simulink library "lib_transmission"  (Simulink 4.1.1)
undefined symbols (not defined in the file or in its folder): fc_map_spd, fc_max_trq, fc_spd_scale, fc_trq_scale, fd_inertia, fd_loss, fd_ratio, gb_inertia, gb_loss_const, gb_loss_input_spd_coeff, gb_loss_input_trq_coeff, gb_loss_output_spd_coeff, gb_loss_output_trq_coeff, gb_map_spd_out, gb_map_trq_in, gb_map_trq_out, gb_ratio, gb_spd_scale, gb_trq_scale, htc_inertia, htc_k_adv, htc_k_adv_coast, htc_max_coast_tr, htc_min_coast_tr, htc_sr, htc_sr_coast, htc_tr, htc_tr_coast, mc_map_spd, mc_max_trq, mc_overtrq_factor, mc_spd_scale, mc_trq_scale, tc_loss, tc_mc_to_fc_ratio, tx_eff_map, tx_map_spd, tx_map_trq, tx_pg_r, tx_pg_s, vc_idle_spd, vc_launch_spd
libraries: lib_transmission x2
(part 1 of 3)
settings Model: LastModifiedBy=tmarkel
settings Model: ModifiedComment=|
  | tmarkel -- Fri Sep 20 16:05:52 2002 -- Version 1.102
  | modified Pout/Pin calc block - moved !=0 check to before bombproof block; value after bombproof is never zero
  | 
  | there are still some issues with this calculation to be resolved at a later date
settings Model: ModifiedHistory=|
  | tmarkel -- Fri Sep 20 16:05:52 2002 -- Version 1.102
  | modified Pout/Pin calc block - moved !=0 check to before bombproof block; value after bombproof is never zero
  | 
  | there are still some issues with this calculation to be resolved at a later date
  | 
  | 
  | tmarkel -- Fri Sep 20 14:16:55 2002 -- Version 1.101
  | changed t loss when tx_eff=0 to be the total torque in request
  | 
  | abrooker -- Fri May 24 14:07:33 2002 -- Version 1.100
  | 
  | mokeefe -- Thu Apr 18 08:38:43 2002 -- Version 1.99
  | saving the model:
  | o "without the model browser open"
  | o with only top-level screen visible
  | o with "fit to view" enabled
  | o with "status bar" off and "toolbar" off
  | o with "prompt to update model history with each save" on

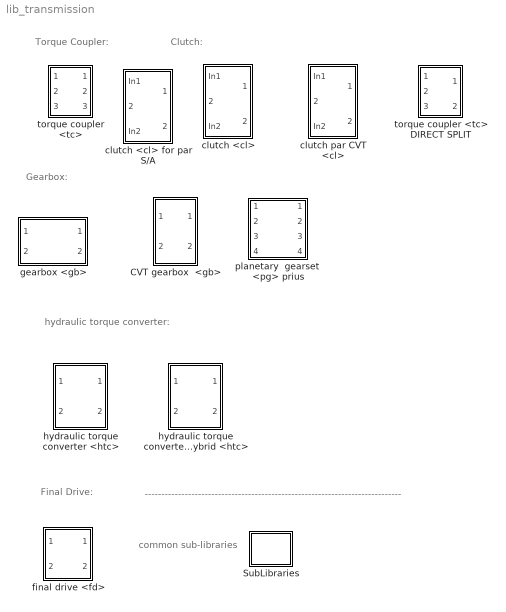
== system lib_transmission ==
  note: Torque Coupler:
  note: Gearbox:
  note: Clutch:
  note: hydraulic torque converter:
  note: Final Drive:
  note: -----------------------------------------------------------------------------
  note: common
      | sub-libraries
  CVT gearbox  <gb> : Subsystem
      settings: RTWFcnNameOpts=Auto  RTWFileNameOpts=Auto
  SubLibraries : Subsystem
      settings: RTWFcnNameOpts=Auto  RTWFileNameOpts=Auto
  clutch <cl> : Subsystem  mask(Clutch){slip_spd=vc_launch_spd, maxtrq=max(fc_max_trq)*fc_trq_scale}
      mask prompts: slip_spd "Input shaft speed when clutch slips (rad/s):"; maxtrq "Maximum torque clutch can transmit:"
      mask help: Clutch for use with ADVISOR 2
      settings: RTWFcnNameOpts=Auto  RTWFileNameOpts=Auto
      mask Help:
      | First input is req'd clutch output torque and speed, muxed together.
      | Second input is clutch state, with 1 => disengaged, 2 => slipping, and 3=> engaged.
      | Third input is available clutch input torque and limited clutch input speed.
      | First output is req'd clutch input torque and speed, muxed together.
      | Second output is available clutch output torque and limited clutch output speed.
      | The logic implemented by this block is as follows:
      |           IF (clutch is disengaged) THEN (req'd input torque=0), (req'd input speed=req'd output speed (the engine control is responsible for computing correct engine spin-down speed)), (avail. output torque=0), (limited output speed=req'd output speed)
      |           IF (clutch is slipping) THEN (req'd input torque=req'd output torque), (req'd input speed=user-defined slip speed), (avail. output torque=avail. input torque), (limited output speed=req'd output speed)
      |           IF (clutch is engaged) THEN (req'd input torque=req'd output torque), (req'd input speed=req'd output speed), (avail. output torque=avail. input torque), (limited output speed=limited input speed)
      | 
      | The clutch will transmit no more than its maximum torque as driving or braking torque.
      mask Display: image(imread('bdi_cl.jpg'))
  clutch <cl> for par S/A : Subsystem  mask(Clutch){slip_spd=vc_launch_spd, maxtrq=max(fc_max_trq)*fc_trq_scale+max(mc_max_trq)*mc_overtrq_factor*mc_trq_scale}
      mask prompts: slip_spd "Input shaft speed when clutch slips (rad/s):"; maxtrq "Maximum torque clutch can transmit:"
      mask help: Clutch for use with ADVISOR 2
      settings: RTWFcnNameOpts=Auto  RTWFileNameOpts=Auto
      mask Help:
      | First input is req'd clutch output torque and speed, muxed together.
      | Second input is clutch state, with 1 => disengaged, 2 => slipping, and 3=> engaged.
      | Third input is available clutch input torque and limited clutch input speed.
      | First output is req'd clutch input torque and speed, muxed together.
      | Second output is available clutch output torque and limited clutch output speed.
      | The logic implemented by this block is as follows:
      |           IF (clutch is disengaged) THEN (req'd input torque=0), (req'd input speed=req'd output speed (the engine control is responsible for computing correct engine spin-down speed)), (avail. output torque=0), (limited output speed=req'd output speed)
      |           IF (clutch is slipping) THEN (req'd input torque=req'd output torque), (req'd input speed=user-defined slip speed), (avail. output torque=avail. input torque), (limited output speed=req'd output speed)
      |           IF (clutch is engaged) THEN (req'd input torque=req'd output torque), (req'd input speed=req'd output speed), (avail. output torque=avail. input torque), (limited output speed=limited input speed)
      | 
      | The clutch will transmit no more than its maximum torque as driving or braking torque.
      mask Display: image(imread('bdi_cl.jpg'))
  clutch par CVT <cl> : Subsystem  mask(Clutch){slip_spd=vc_launch_spd, maxtrq=max(fc_max_trq)*fc_trq_scale+max(mc_max_trq)*mc_trq_scale*mc_overtrq_factor}
      mask prompts: slip_spd "Input shaft speed when clutch slips (rad/s):"; maxtrq "Maximum torque clutch can transmit:"
      mask help: Clutch for use with ADVISOR 2
      settings: RTWFcnNameOpts=Auto  RTWFileNameOpts=Auto
      mask Help:
      | First input is req'd clutch output torque and speed, muxed together.
      | Second input is clutch state, with 1 => disengaged, 2 => slipping, and 3=> engaged.
      | Third input is available clutch input torque and limited clutch input speed.
      | First output is req'd clutch input torque and speed, muxed together.
      | Second output is available clutch output torque and limited clutch output speed.
      | The logic implemented by this block is as follows:
      |           IF (clutch is disengaged) THEN (req'd input torque=0), (req'd input speed=req'd output speed (the engine control is responsible for computing correct engine spin-down speed)), (avail. output torque=0), (limited output speed=req'd output speed)
      |           IF (clutch is slipping) THEN (req'd input torque=req'd output torque), (req'd input speed=user-defined slip speed), (avail. output torque=avail. input torque), (limited output speed=req'd output speed)
      |           IF (clutch is engaged) THEN (req'd input torque=req'd output torque), (req'd input speed=req'd output speed), (avail. output torque=avail. input torque), (limited output speed=limited input speed)
      | 
      | The clutch will transmit no more than its maximum torque as driving or braking torque.
      mask Display: image(imread('bdi_cl.jpg'))
  final drive <fd> : Subsystem
      settings: RTWFcnNameOpts=Auto  RTWFileNameOpts=Auto
      mask Display: image(imread('bdi_fd.jpg'))
  gearbox <gb> : Subsystem
      settings: RTWFcnNameOpts=Auto  RTWFileNameOpts=Auto
      mask Display: image(imread('bdi_gb.jpg'))
  hydraulic torque converter <htc> : Subsystem
      settings: RTWFcnNameOpts=Auto  RTWFileNameOpts=Auto
      mask Display: image(imread('bdi_htc.jpg'))
  hydraulic torque converter for  parallel hybrid <htc> : Subsystem
      settings: RTWFcnNameOpts=Auto  RTWFileNameOpts=Auto
      mask Display: image(imread('bdi_htc.jpg'))
  planetary  gearset  <pg> prius : Subsystem
      settings: RTWFcnNameOpts=Auto  RTWFileNameOpts=Auto
      mask Display: image(imread('bdi_psplit.jpg'))
  torque coupler <tc> : Subsystem
      settings: RTWFcnNameOpts=Auto  RTWFileNameOpts=Auto
      mask Display: image(imread('bdi_tc.jpg'))
  torque coupler <tc> DIRECT SPLIT : Subsystem
      settings: RTWFcnNameOpts=Auto  RTWFileNameOpts=Auto
      mask Display: image(imread('bdi_tc.jpg'))

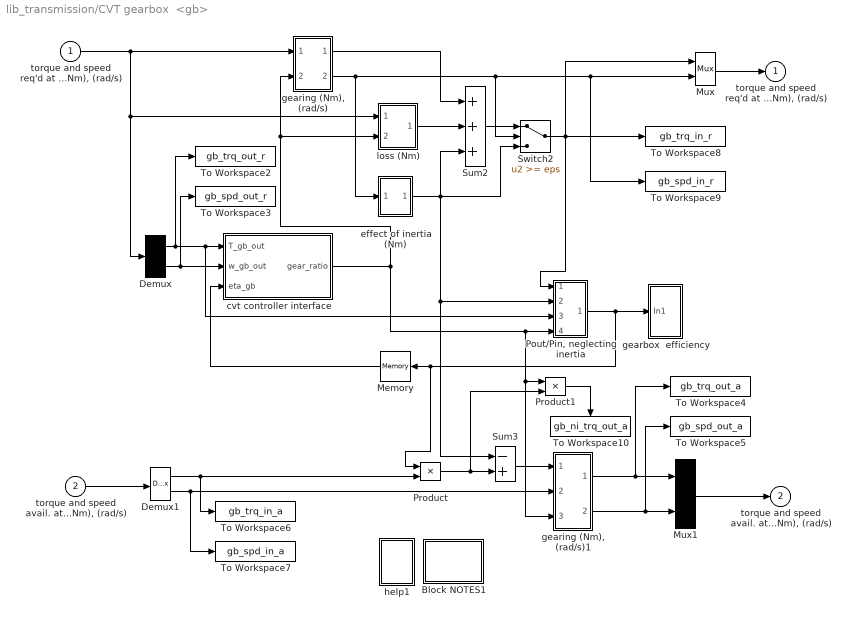
== system lib_transmission/CVT gearbox  <gb> ==
  "torque and speed req'd at output side of cvt (Nm), (rad/s)" : Inport  Port=1  LatchInput=off
  "torque and speed avail. at input side of cvt (Nm), (rad/s)" : Inport  Port=2  LatchInput=off
  Block NOTES1 : Subsystem
      settings: RTWFcnNameOpts=Auto  RTWFileNameOpts=Auto
      mask Display: disp('Block\nNOTES')
  Demux : Demux  Outputs=2  BusSelectionMode=off
  Demux1 : Demux  Outputs=2  BusSelectionMode=off
  Memory : Memory  Orientation=left  X0=0.9  InheritSampleTime=off
      settings: RTWStateStorageClass=Auto
  Mux : Mux  Inputs=2
      settings: DisplayOption=none
  Mux1 : Mux  Inputs=2
      settings: DisplayOption=none
  "Pout/Pin, neglecting inertia" : Subsystem
      settings: RTWFcnNameOpts=Auto  RTWFileNameOpts=Auto
  Product : Product  Inputs=2  Multiplication=Element-wise(.*)  SaturateOnIntegerOverflow=on
  Product1 : Product  Inputs=2  Multiplication=Element-wise(.*)  SaturateOnIntegerOverflow=on
  Sum2 : Sum  Inputs=+++  SaturateOnIntegerOverflow=on
  Sum3 : Sum  Inputs=-+  SaturateOnIntegerOverflow=on
  Switch2 : Switch  Threshold=eps
  To Workspace10 : ToWorkspace  VariableName=gb_ni_trq_out_a  SampleTime=-1  SaveFormat=Array
      settings: Orientation=down
  To Workspace2 : ToWorkspace  VariableName=gb_trq_out_r  SampleTime=-1  SaveFormat=Array
  To Workspace3 : ToWorkspace  VariableName=gb_spd_out_r  SampleTime=-1  SaveFormat=Array
  To Workspace4 : ToWorkspace  VariableName=gb_trq_out_a  SampleTime=-1  SaveFormat=Array
  To Workspace5 : ToWorkspace  VariableName=gb_spd_out_a  SampleTime=-1  SaveFormat=Array
  To Workspace6 : ToWorkspace  VariableName=gb_trq_in_a  SampleTime=-1  SaveFormat=Array
  To Workspace7 : ToWorkspace  VariableName=gb_spd_in_a  SampleTime=-1  SaveFormat=Array
  To Workspace8 : ToWorkspace  VariableName=gb_trq_in_r  SampleTime=-1  SaveFormat=Array
  To Workspace9 : ToWorkspace  VariableName=gb_spd_in_r  SampleTime=-1  SaveFormat=Array
  cvt controller interface : Subsystem
      settings: RTWFcnNameOpts=Auto  RTWFileNameOpts=Auto
  effect of inertia (Nm) : Subsystem
      settings: RTWFcnNameOpts=Auto  RTWFileNameOpts=Auto
  gearbox  efficiency : Subsystem
      settings: RTWFcnNameOpts=Auto  RTWFileNameOpts=Auto
  "gearing (Nm), (rad/s)" : Subsystem
      settings: RTWFcnNameOpts=Auto  RTWFileNameOpts=Auto
  "gearing (Nm), (rad/s)1" : Subsystem
      settings: RTWFcnNameOpts=Auto  RTWFileNameOpts=Auto
  help1 : Subsystem
      settings: OpenFcn=web(['file:\\\' which('cvt.htm')]);  RTWFcnNameOpts=Auto  RTWFileNameOpts=Auto
      mask Display: image(imread('doc_man.jpg'))
  loss (Nm) : Subsystem
      settings: RTWFcnNameOpts=Auto  RTWFileNameOpts=Auto
  "torque and speed req'd at input side of cvt (Nm), (rad/s)" : Outport  Port=1  InitialOutput=0
  "torque and speed avail. at output side of cvt (Nm), (rad/s)" : Outport  Port=2  InitialOutput=0
  wires:
  "Pout/Pin, neglecting inertia"/1(Pout/Pin) -> gearbox  efficiency/1(In1), Product/1, Memory/1
  Switch2/1 -> "Pout/Pin, neglecting inertia"/1(Tin), Mux/1, To Workspace8/1
  Sum2/1 -> Switch2/1
  Mux1/1 -> "torque and speed avail. at output side of cvt (Nm), (rad/s)"/1
  Sum3/1 -> "gearing (Nm), (rad/s)1"/1(input shaft torque (Nm))
  "torque and speed avail. at input side of cvt (Nm), (rad/s)"/1 -> Demux1/1
  Mux/1 -> "torque and speed req'd at input side of cvt (Nm), (rad/s)"/1
  "gearing (Nm), (rad/s)"/1(input shaft torque (Nm)) -> Sum2/1
  "gearing (Nm), (rad/s)"/2(input shaft speed (rad/s)) -> Switch2/2, Mux/2, To Workspace9/1, effect of inertia (Nm)/1(gb input speed (rad/s))
  effect of inertia (Nm)/1(drag torque (Nm)) -> Switch2/3, Sum2/3, Sum3/1, "Pout/Pin, neglecting inertia"/2(Tinertia)
  "torque and speed req'd at output side of cvt (Nm), (rad/s)"/1 -> "gearing (Nm), (rad/s)"/1("output shaft torque and speed  (Nm), (rad/s)"), loss (Nm)/1("output torque and speed (Nm), (rad/s)"), Demux/1
  Demux/2 -> cvt controller interface/2(w_gb_out), To Workspace3/1
  Demux/1 -> cvt controller interface/1(T_gb_out), "Pout/Pin, neglecting inertia"/3(Tout), To Workspace2/1
  "gearing (Nm), (rad/s)1"/2(output shaft speed (rad/s)) -> Mux1/2, To Workspace5/1
  "gearing (Nm), (rad/s)1"/1(output shaft torque (Nm)) -> Mux1/1, To Workspace4/1
  Demux1/1 -> Product/2, To Workspace6/1
  Demux1/2 -> "gearing (Nm), (rad/s)1"/2(input shaft speed (rad/s)), To Workspace7/1
  loss (Nm)/1(loss torque at input shaft (Nm)) -> Sum2/2
  cvt controller interface/1(gear_ratio) -> loss (Nm)/2(pulley ratio), "gearing (Nm), (rad/s)"/2(gear ratio), "Pout/Pin, neglecting inertia"/4(gear ratio), "gearing (Nm), (rad/s)1"/3(gear ratio), Product1/1
  Memory/1 -> cvt controller interface/3(eta_gb)
  Product1/1 -> To Workspace10/1
  Product/1 -> Sum3/2, Product1/2

== system lib_transmission/SubLibraries ==
  note: Trq and Spd at Output
      | (Nm) and (rad/s)
  note: Gear Ratio
      | (input spd/output spd)
  note: Trq loss
      | at input (Nm)
  note: gear ratio
      | (input/output spd)
  note: gear (1st, 2nd, etc.)
  note: data needs:
      | gb_ratio
  note: Below is the loss block for a gear box based
      | on loss equation--used with ADVISOR v. 3.1 and below
  note: X_lookup
  note: Y_lookup
  note: Z_discrete value
  note: looked up value
  note: X_lookup
  note: Y_lookup
  note: Z_discrete value
  note: looked up value
  3D discrete lookup table : Subsystem  mask{tx_map_spd=tx_map_spd, tx_map_trq=tx_map_trq, tx_eff_map=tx_eff_map}
      mask prompts: tx_map_spd "Row Lookup"; tx_map_trq "Column Lookup"; tx_eff_map "Lookup Matrix"
      settings: RTWFcnNameOpts=Auto  RTWFileNameOpts=Auto
  3D discrete lookup table (sfun) : Subsystem  mask{tx_map_spd=tx_map_spd, tx_map_trq=tx_map_trq, tx_eff_map=tx_eff_map}
      mask prompts: tx_map_spd "Row Lookup"; tx_map_trq "Column Lookup"; tx_eff_map "Lookup Matrix"
      settings: RTWFcnNameOpts=Auto  RTWFileNameOpts=Auto
  "gear determination (e.g., 1st gear, 2nd, etc.)" : Subsystem
      settings: RTWFcnNameOpts=Auto  RTWFileNameOpts=Auto
  loss (Nm) : Subsystem  mask{tx_eff_map=tx_eff_map, tx_map_trq=tx_map_trq, tx_map_spd=tx_map_spd, gb_spd_scale=gb_spd_scale, gb_trq_scale=gb_trq_scale}
      mask prompts: tx_eff_map "table of efficiency values (spd rad/s, trq Nm)"; tx_map_trq "vector of output torque values for lookup table (Nm)"; tx_map_spd "vector of output speeds for lookup table (rad/s)"; gb_spd_scale "Speed scale for the transmission gear box"; gb_trq_scale "Torque scale for the transmission gear box"
      settings: RTWFcnNameOpts=Auto  RTWFileNameOpts=Auto
  loss (Nm) old methodology : Subsystem
      settings: RTWFcnNameOpts=Auto  RTWFileNameOpts=Auto
  notes on  3D discrete lookup table : Subsystem
      settings: RTWFcnNameOpts=Auto  RTWFileNameOpts=Auto
  notes on  loss (Nm) : Subsystem
      settings: RTWFcnNameOpts=Auto  RTWFileNameOpts=Auto

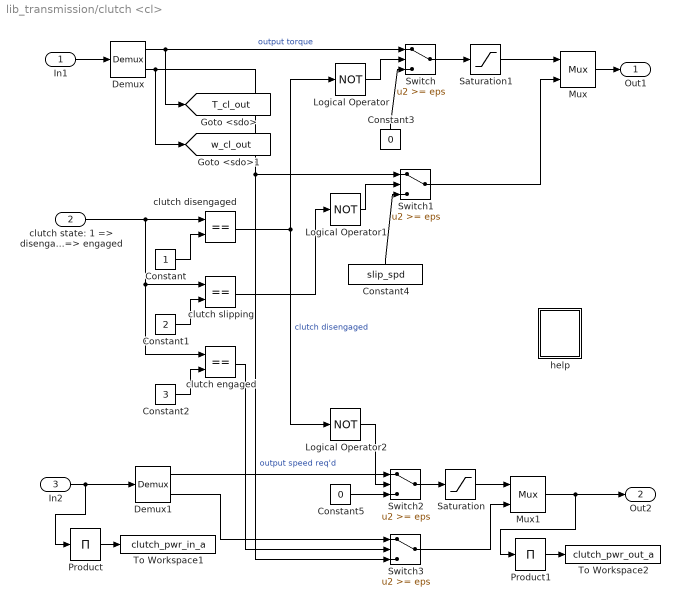
== system lib_transmission/clutch <cl> ==
  In1 : Inport  Port=1  LatchInput=off
  clutch state: 1 => disengaged 2 => slipping 3 => engaged : Inport  Port=2  LatchInput=off
  In2 : Inport  Port=3  LatchInput=off
  Constant : Constant  Value=1
  Constant1 : Constant  Value=2
  Constant2 : Constant  Value=3
  Constant3 : Constant  Orientation=up  Value=0
  Constant4 : Constant  Orientation=up  Value=slip_spd
  Constant5 : Constant  Value=0
  Demux : Demux  Outputs=2  BusSelectionMode=off
  Demux1 : Demux  Outputs=2  BusSelectionMode=off
  Logical Operator : Logic  Operator=NOT  Inputs=1
  Logical Operator1 : Logic  Operator=NOT  Inputs=1
  Logical Operator2 : Logic  Operator=NOT  Inputs=1
  Mux : Mux  Inputs=2
      settings: DisplayOption=none
  Mux1 : Mux  Inputs=2
      settings: DisplayOption=none
  Product : Product  Inputs=1  Multiplication=Element-wise(.*)  SaturateOnIntegerOverflow=on
  Product1 : Product  Inputs=1  Multiplication=Element-wise(.*)  SaturateOnIntegerOverflow=on
  Saturation : Saturate  UpperLimit=maxtrq  LowerLimit=-maxtrq  LinearizeAsGain=on
  Saturation1 : Saturate  UpperLimit=maxtrq  LowerLimit=-maxtrq  LinearizeAsGain=on
  Switch{,1..3} (4 alike) : Switch  Threshold=eps
  To Workspace1 : ToWorkspace  VariableName=clutch_pwr_in_a  SampleTime=-1  SaveFormat=Array
  To Workspace2 : ToWorkspace  VariableName=clutch_pwr_out_a  SampleTime=-1  SaveFormat=Array
  clutch disengaged : RelationalOperator  Operator===
  clutch engaged : RelationalOperator  Operator===
  clutch slipping : RelationalOperator  Operator===
  help : Subsystem
      settings: OpenFcn=web(['file:\\\' which('clutch.htm')]);  RTWFcnNameOpts=Auto  RTWFileNameOpts=Auto
      mask Display: image(imread('doc_man.jpg'))
  Out1 : Outport  Port=1
  Out2 : Outport  Port=2
  tag scope: T_cl_out=global, w_cl_out=global
  wires:
  Saturation1/1 -> Mux/1
  Switch/1 -> Saturation1/1
  Saturation/1 -> Mux1/1
  Switch2/1 -> Saturation/1
  Constant/1 -> clutch disengaged/2
  Constant1/1 -> clutch slipping/2
  clutch state: 1 => disengaged 2 => slipping 3 => engaged/1 -> clutch disengaged/1, clutch slipping/1, clutch engaged/1
  In1/1 -> Demux/1
  Mux/1 -> Out1/1
  Constant2/1 -> clutch engaged/2
  clutch slipping/1 -> Logical Operator1/1
  clutch disengaged/1 -> Logical Operator/1, Logical Operator2/1  "clutch disengaged"
  Logical Operator/1 -> Switch/2
  Constant3/1 -> Switch/3
  Logical Operator1/1 -> Switch1/2
  Constant4/1 -> Switch1/3
  Switch1/1 -> Mux/2
  Demux1/1 -> Switch2/1
  Logical Operator2/1 -> Switch2/2
  Constant5/1 -> Switch2/3
  Demux1/2 -> Switch3/1
  Switch3/1 -> Mux1/2
  clutch engaged/1 -> Switch3/2
  Demux/1 -> Switch/1, [T_cl_out]  "output torque"
  Demux/2 -> Switch1/1, Switch3/3, [w_cl_out]  "output speed req'd"
  In2/1 -> Demux1/1, Product/1
  Product/1 -> To Workspace1/1
  Product1/1 -> To Workspace2/1
  Mux1/1 -> Out2/1, Product1/1

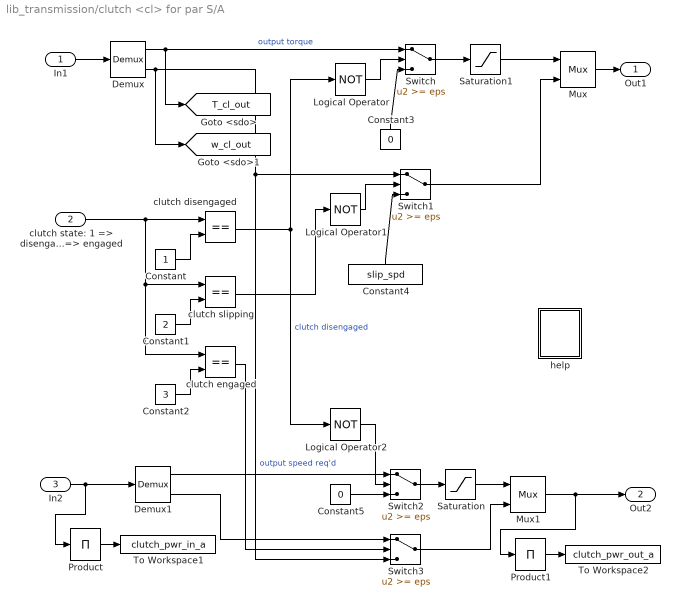
== system lib_transmission/clutch <cl> for par S/A ==
  In1 : Inport  Port=1  LatchInput=off
  clutch state: 1 => disengaged 2 => slipping 3 => engaged : Inport  Port=2  LatchInput=off
  In2 : Inport  Port=3  LatchInput=off
  Constant : Constant  Value=1
  Constant1 : Constant  Value=2
  Constant2 : Constant  Value=3
  Constant3 : Constant  Orientation=up  Value=0
  Constant4 : Constant  Orientation=up  Value=slip_spd
  Constant5 : Constant  Value=0
  Demux : Demux  Outputs=2  BusSelectionMode=off
  Demux1 : Demux  Outputs=2  BusSelectionMode=off
  Logical Operator : Logic  Operator=NOT  Inputs=1
  Logical Operator1 : Logic  Operator=NOT  Inputs=1
  Logical Operator2 : Logic  Operator=NOT  Inputs=1
  Mux : Mux  Inputs=2
      settings: DisplayOption=none
  Mux1 : Mux  Inputs=2
      settings: DisplayOption=none
  Product : Product  Inputs=1  Multiplication=Element-wise(.*)  SaturateOnIntegerOverflow=on
  Product1 : Product  Inputs=1  Multiplication=Element-wise(.*)  SaturateOnIntegerOverflow=on
  Saturation : Saturate  UpperLimit=maxtrq  LowerLimit=-maxtrq  LinearizeAsGain=on
  Saturation1 : Saturate  UpperLimit=maxtrq  LowerLimit=-maxtrq  LinearizeAsGain=on
  Switch{,1..3} (4 alike) : Switch  Threshold=eps
  To Workspace1 : ToWorkspace  VariableName=clutch_pwr_in_a  SampleTime=-1  SaveFormat=Array
  To Workspace2 : ToWorkspace  VariableName=clutch_pwr_out_a  SampleTime=-1  SaveFormat=Array
  clutch disengaged : RelationalOperator  Operator===
  clutch engaged : RelationalOperator  Operator===
  clutch slipping : RelationalOperator  Operator===
  help : Subsystem
      settings: OpenFcn=web(['file:\\\' which('clutch.htm')]);  RTWFcnNameOpts=Auto  RTWFileNameOpts=Auto
      mask Display: image(imread('doc_man.jpg'))
  Out1 : Outport  Port=1
  Out2 : Outport  Port=2
  tag scope: T_cl_out=global, w_cl_out=global
  wires:
  Mux1/1 -> Product1/1, Out2/1
  Product1/1 -> To Workspace2/1
  Product/1 -> To Workspace1/1
  In2/1 -> Product/1, Demux1/1
  Demux/2 -> [w_cl_out], Switch3/3, Switch1/1  "output speed req'd"
  Demux/1 -> [T_cl_out], Switch/1  "output torque"
  clutch engaged/1 -> Switch3/2
  Switch3/1 -> Mux1/2
  Demux1/2 -> Switch3/1
  Constant5/1 -> Switch2/3
  Logical Operator2/1 -> Switch2/2
  Demux1/1 -> Switch2/1
  Switch1/1 -> Mux/2
  Constant4/1 -> Switch1/3
  Logical Operator1/1 -> Switch1/2
  Constant3/1 -> Switch/3
  Logical Operator/1 -> Switch/2
  clutch disengaged/1 -> Logical Operator2/1, Logical Operator/1  "clutch disengaged"
  clutch slipping/1 -> Logical Operator1/1
  Constant2/1 -> clutch engaged/2
  Mux/1 -> Out1/1
  In1/1 -> Demux/1
  clutch state: 1 => disengaged 2 => slipping 3 => engaged/1 -> clutch engaged/1, clutch slipping/1, clutch disengaged/1
  Constant1/1 -> clutch slipping/2
  Constant/1 -> clutch disengaged/2
  Switch2/1 -> Saturation/1
  Saturation/1 -> Mux1/1
  Switch/1 -> Saturation1/1
  Saturation1/1 -> Mux/1

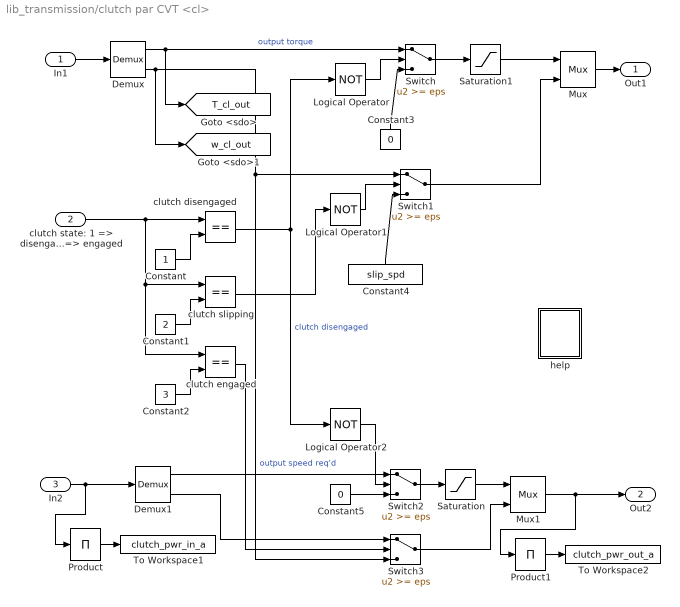
== system lib_transmission/clutch par CVT <cl> ==
  In1 : Inport  Port=1  LatchInput=off
  clutch state: 1 => disengaged 2 => slipping 3 => engaged : Inport  Port=2  LatchInput=off
  In2 : Inport  Port=3  LatchInput=off
  Constant : Constant  Value=1
  Constant1 : Constant  Value=2
  Constant2 : Constant  Value=3
  Constant3 : Constant  Orientation=up  Value=0
  Constant4 : Constant  Orientation=up  Value=slip_spd
  Constant5 : Constant  Value=0
  Demux : Demux  Outputs=2  BusSelectionMode=off
  Demux1 : Demux  Outputs=2  BusSelectionMode=off
  Logical Operator : Logic  Operator=NOT  Inputs=1
  Logical Operator1 : Logic  Operator=NOT  Inputs=1
  Logical Operator2 : Logic  Operator=NOT  Inputs=1
  Mux : Mux  Inputs=2
      settings: DisplayOption=none
  Mux1 : Mux  Inputs=2
      settings: DisplayOption=none
  Product : Product  Inputs=1  Multiplication=Element-wise(.*)  SaturateOnIntegerOverflow=on
  Product1 : Product  Inputs=1  Multiplication=Element-wise(.*)  SaturateOnIntegerOverflow=on
  Saturation : Saturate  UpperLimit=maxtrq  LowerLimit=-maxtrq  LinearizeAsGain=on
  Saturation1 : Saturate  UpperLimit=maxtrq  LowerLimit=-maxtrq  LinearizeAsGain=on
  Switch{,1..3} (4 alike) : Switch  Threshold=eps
  To Workspace1 : ToWorkspace  VariableName=clutch_pwr_in_a  SampleTime=-1  SaveFormat=Array
  To Workspace2 : ToWorkspace  VariableName=clutch_pwr_out_a  SampleTime=-1  SaveFormat=Array
  clutch disengaged : RelationalOperator  Operator===
  clutch engaged : RelationalOperator  Operator===
  clutch slipping : RelationalOperator  Operator===
  help : Subsystem
      settings: OpenFcn=web(['file:\\\' which('clutch.htm')]);  RTWFcnNameOpts=Auto  RTWFileNameOpts=Auto
      mask Display: image(imread('doc_man.jpg'))
  Out1 : Outport  Port=1
  Out2 : Outport  Port=2
  tag scope: T_cl_out=global, w_cl_out=global
  wires:
  Saturation1/1 -> Mux/1
  Switch/1 -> Saturation1/1
  Saturation/1 -> Mux1/1
  Switch2/1 -> Saturation/1
  Constant/1 -> clutch disengaged/2
  Constant1/1 -> clutch slipping/2
  clutch state: 1 => disengaged 2 => slipping 3 => engaged/1 -> clutch disengaged/1, clutch slipping/1, clutch engaged/1
  In1/1 -> Demux/1
  Mux/1 -> Out1/1
  Constant2/1 -> clutch engaged/2
  clutch slipping/1 -> Logical Operator1/1
  clutch disengaged/1 -> Logical Operator/1, Logical Operator2/1  "clutch disengaged"
  Logical Operator/1 -> Switch/2
  Constant3/1 -> Switch/3
  Logical Operator1/1 -> Switch1/2
  Constant4/1 -> Switch1/3
  Switch1/1 -> Mux/2
  Demux1/1 -> Switch2/1
  Logical Operator2/1 -> Switch2/2
  Constant5/1 -> Switch2/3
  Demux1/2 -> Switch3/1
  Switch3/1 -> Mux1/2
  clutch engaged/1 -> Switch3/2
  Demux/1 -> Switch/1, [T_cl_out]  "output torque"
  Demux/2 -> Switch1/1, Switch3/3, [w_cl_out]  "output speed req'd"
  In2/1 -> Demux1/1, Product/1
  Product/1 -> To Workspace1/1
  Product1/1 -> To Workspace2/1
  Mux1/1 -> Out2/1, Product1/1

== system lib_transmission/final drive <fd> ==
  "torque and speed req'd at output side of final drive (Nm), (rad/s)" : Inport  Port=1  LatchInput=off
  "torque and speed avail. at input side of final drive (Nm), (rad/s)" : Inport  Port=2  LatchInput=off
  Block NOTES : Subsystem
      settings: RTWFcnNameOpts=Auto  RTWFileNameOpts=Auto
      mask Display: disp('Block\nNOTES')
  Demux : Demux  Outputs=2  BusSelectionMode=off
  Demux1 : Demux  Outputs=2  BusSelectionMode=off
  Gain : Gain  Gain=fd_ratio  Multiplication=Element-wise(K.*u)  SaturateOnIntegerOverflow=on
  Gain1 : Gain  Gain=1/fd_ratio  Multiplication=Element-wise(K.*u)  SaturateOnIntegerOverflow=on
  Gain2 : Gain  Gain=fd_ratio  Multiplication=Element-wise(K.*u)  SaturateOnIntegerOverflow=on
  Gain3 : Gain  Gain=1/fd_ratio  Multiplication=Element-wise(K.*u)  SaturateOnIntegerOverflow=on
  Mux : Mux  Inputs=2
      settings: DisplayOption=none
  Mux1 : Mux  Inputs=2
      settings: DisplayOption=none
  Sum1 : Sum  Inputs=--+  SaturateOnIntegerOverflow=on
  Sum2 : Sum  Inputs=+++  SaturateOnIntegerOverflow=on
  To Workspace2 : ToWorkspace  VariableName=fd_trq_out_r  SampleTime=-1  SaveFormat=Array
  To Workspace3 : ToWorkspace  VariableName=fd_spd_out_r  SampleTime=-1  SaveFormat=Array
  To Workspace4 : ToWorkspace  VariableName=fd_trq_in_r  SampleTime=-1  SaveFormat=Array
  To Workspace5 : ToWorkspace  VariableName=fd_spd_in_r  SampleTime=-1  SaveFormat=Array
  To Workspace6 : ToWorkspace  VariableName=fd_trq_in_a  SampleTime=-1  SaveFormat=Array
  To Workspace7 : ToWorkspace  VariableName=fd_spd_in_a  SampleTime=-1  SaveFormat=Array
  To Workspace8 : ToWorkspace  VariableName=fd_trq_out_a  SampleTime=-1  SaveFormat=Array
  To Workspace9 : ToWorkspace  VariableName=fd_spd_out_a  SampleTime=-1  SaveFormat=Array
  effect of inertia (Nm) : Subsystem
      settings: RTWFcnNameOpts=Auto  RTWFileNameOpts=Auto
  help : Subsystem
      settings: OpenFcn=web(['file:\\\' which('wheel_axle.htm')]);  RTWFcnNameOpts=Auto  RTWFileNameOpts=Auto
      mask Display: image(imread('doc_man.jpg'))
  loss (Nm) : Subsystem
      settings: RTWFcnNameOpts=Auto  RTWFileNameOpts=Auto
  "torque and speed req'd at input side of final drive (Nm), (rad/s)" : Outport  Port=1  InitialOutput=0
  "torque and speed avail. at output side of final drive (Nm), (rad/s)" : Outport  Port=2  InitialOutput=0
  wires:
  Sum1/1 -> Gain2/1
  "torque and speed avail. at input side of final drive (Nm), (rad/s)"/1 -> Demux1/1
  Mux1/1 -> "torque and speed avail. at output side of final drive (Nm), (rad/s)"/1
  loss (Nm)/1(drag torque (Nm)) -> Sum1/1, Sum2/2
  effect of inertia (Nm)/1(drag torque (Nm)) -> Sum1/2, Sum2/3
  Gain/1 -> loss (Nm)/1(fd output speed (rad/s)), effect of inertia (Nm)/1(fd input speed (rad/s)), Mux/2, To Workspace5/1
  Gain1/1 -> Sum2/1
  "torque and speed req'd at output side of final drive (Nm), (rad/s)"/1 -> Demux/1
  Mux/1 -> "torque and speed req'd at input side of final drive (Nm), (rad/s)"/1
  Demux/1 -> Gain1/1, To Workspace2/1
  Demux/2 -> Gain/1, To Workspace3/1
  Sum2/1 -> Mux/1, To Workspace4/1
  Demux1/1 -> Sum1/3, To Workspace6/1
  Demux1/2 -> Gain3/1, To Workspace7/1
  Gain3/1 -> Mux1/2, To Workspace9/1
  Gain2/1 -> Mux1/1, To Workspace8/1

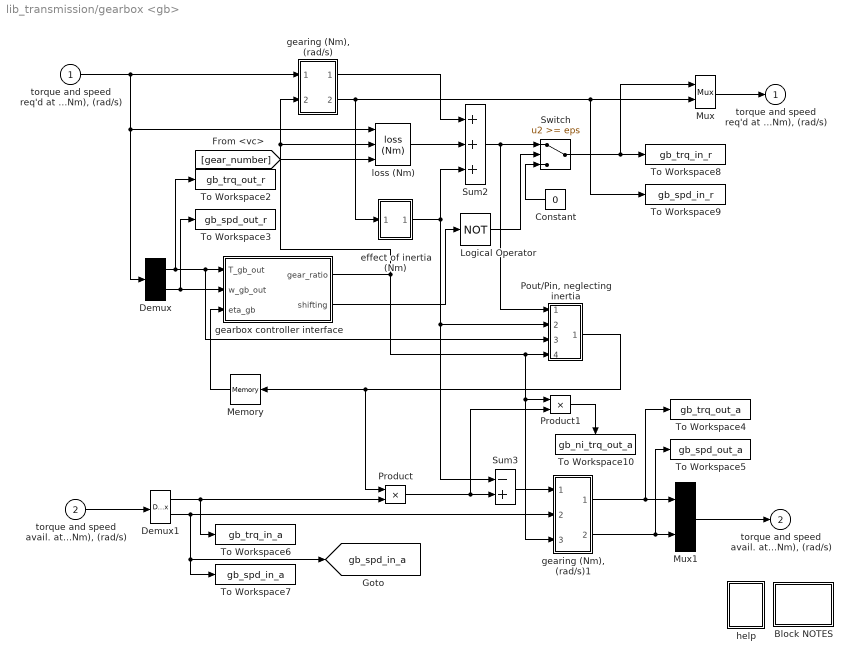
== system lib_transmission/gearbox <gb> ==
  "torque and speed req'd at output side of gearbox (Nm), (rad/s)" : Inport  Port=1  LatchInput=off
  "torque and speed avail. at input side of gearbox (Nm), (rad/s)" : Inport  Port=2  LatchInput=off
  Block NOTES : Subsystem
      settings: RTWFcnNameOpts=Auto  RTWFileNameOpts=Auto
      mask Display: disp('Block\nNOTES')
  Constant : Constant  Orientation=left  Value=0
  Demux : Demux  Outputs=2  BusSelectionMode=off
  Demux1 : Demux  Outputs=2  BusSelectionMode=off
  Logical Operator : Logic  Operator=NOT  Inputs=1
  Memory : Memory  Orientation=left  X0=0  InheritSampleTime=off
      settings: RTWStateStorageClass=Auto
  Mux : Mux  Inputs=2
      settings: DisplayOption=none
  Mux1 : Mux  Inputs=2
      settings: DisplayOption=none
  "Pout/Pin, neglecting inertia" : Subsystem
      settings: RTWFcnNameOpts=Auto  RTWFileNameOpts=Auto
  Product : Product  Inputs=2  Multiplication=Element-wise(.*)  SaturateOnIntegerOverflow=on
  Product1 : Product  Inputs=2  Multiplication=Element-wise(.*)  SaturateOnIntegerOverflow=on
  Sum2 : Sum  Inputs=+++  SaturateOnIntegerOverflow=on
  Sum3 : Sum  Inputs=-+  SaturateOnIntegerOverflow=on
  Switch : Switch  Threshold=eps
  To Workspace10 : ToWorkspace  VariableName=gb_ni_trq_out_a  SampleTime=-1  SaveFormat=Array
      settings: Orientation=down
  To Workspace2 : ToWorkspace  VariableName=gb_trq_out_r  SampleTime=-1  SaveFormat=Array
  To Workspace3 : ToWorkspace  VariableName=gb_spd_out_r  SampleTime=-1  SaveFormat=Array
  To Workspace4 : ToWorkspace  VariableName=gb_trq_out_a  SampleTime=-1  SaveFormat=Array
  To Workspace5 : ToWorkspace  VariableName=gb_spd_out_a  SampleTime=-1  SaveFormat=Array
  To Workspace6 : ToWorkspace  VariableName=gb_trq_in_a  SampleTime=-1  SaveFormat=Array
  To Workspace7 : ToWorkspace  VariableName=gb_spd_in_a  SampleTime=-1  SaveFormat=Array
  To Workspace8 : ToWorkspace  VariableName=gb_trq_in_r  SampleTime=-1  SaveFormat=Array
  To Workspace9 : ToWorkspace  VariableName=gb_spd_in_r  SampleTime=-1  SaveFormat=Array
  effect of inertia (Nm) : Subsystem
      settings: RTWFcnNameOpts=Auto  RTWFileNameOpts=Auto
  gearbox controller interface : Subsystem
      settings: RTWFcnNameOpts=Auto  RTWFileNameOpts=Auto
  "gearing (Nm), (rad/s)" : Subsystem
      settings: RTWFcnNameOpts=Auto  RTWFileNameOpts=Auto
  "gearing (Nm), (rad/s)1" : Subsystem
      settings: RTWFcnNameOpts=Auto  RTWFileNameOpts=Auto
  help : Subsystem
      settings: OpenFcn=web(['file:\\\' which('gearbox.htm')]);  RTWFcnNameOpts=Auto  RTWFileNameOpts=Auto
      mask Display: image(imread('doc_man.jpg'))
  loss (Nm) : lib_transmission/SubLibraries/loss (Nm)  tx_eff_map=tx_eff_map  tx_map_trq=tx_map_trq  tx_map_spd=tx_map_spd  gb_spd_scale=gb_spd_scale  gb_trq_scale=gb_trq_scale
  "torque and speed req'd at input side of gearbox (Nm), (rad/s)" : Outport  Port=1  InitialOutput=0
  "torque and speed avail. at output side of gearbox (Nm), (rad/s)" : Outport  Port=2  InitialOutput=0
  tag scope: gb_spd_in_a=global
  wires:
  gearbox controller interface/1(gear_ratio) -> "Pout/Pin, neglecting inertia"/4(gear ratio), "gearing (Nm), (rad/s)1"/3(gear ratio), Product1/1, "gearing (Nm), (rad/s)"/2(gear ratio), loss (Nm)/2
  loss (Nm)/1 -> Sum2/2
  Constant/1 -> Switch/3
  Switch/1 -> Mux/1, To Workspace8/1
  Logical Operator/1 -> Switch/2
  gearbox controller interface/2(shifting) -> Logical Operator/1
  Sum2/1 -> Switch/1, "Pout/Pin, neglecting inertia"/1(Tin)
  Demux1/2 -> [gb_spd_in_a], To Workspace7/1, "gearing (Nm), (rad/s)1"/2(input shaft speed (rad/s))
  Demux1/1 -> To Workspace6/1, Product/2
  "gearing (Nm), (rad/s)1"/1(output shaft torque (Nm)) -> To Workspace4/1, Mux1/1
  "gearing (Nm), (rad/s)1"/2(output shaft speed (rad/s)) -> To Workspace5/1, Mux1/2
  Demux/1 -> To Workspace2/1, "Pout/Pin, neglecting inertia"/3(Tout), gearbox controller interface/1(T_gb_out)
  Demux/2 -> To Workspace3/1, gearbox controller interface/2(w_gb_out)
  "torque and speed req'd at output side of gearbox (Nm), (rad/s)"/1 -> Demux/1, loss (Nm)/1, "gearing (Nm), (rad/s)"/1("output shaft torque and speed  (Nm), (rad/s)")
  effect of inertia (Nm)/1(drag torque (Nm)) -> "Pout/Pin, neglecting inertia"/2(Tinertia), Sum3/1, Sum2/3
  "gearing (Nm), (rad/s)"/2(input shaft speed (rad/s)) -> To Workspace9/1, Mux/2, effect of inertia (Nm)/1(gb input speed (rad/s))
  "gearing (Nm), (rad/s)"/1(input shaft torque (Nm)) -> Sum2/1
  Mux/1 -> "torque and speed req'd at input side of gearbox (Nm), (rad/s)"/1
  Memory/1 -> gearbox controller interface/3(eta_gb)
  "Pout/Pin, neglecting inertia"/1(Pout/Pin) -> Product/1, Memory/1
  "torque and speed avail. at input side of gearbox (Nm), (rad/s)"/1 -> Demux1/1
  Sum3/1 -> "gearing (Nm), (rad/s)1"/1(input shaft torque (Nm))
  Mux1/1 -> "torque and speed avail. at output side of gearbox (Nm), (rad/s)"/1
  Product/1 -> Sum3/2, Product1/2
  Product1/1 -> To Workspace10/1
  [gear_number] -> loss (Nm)/3

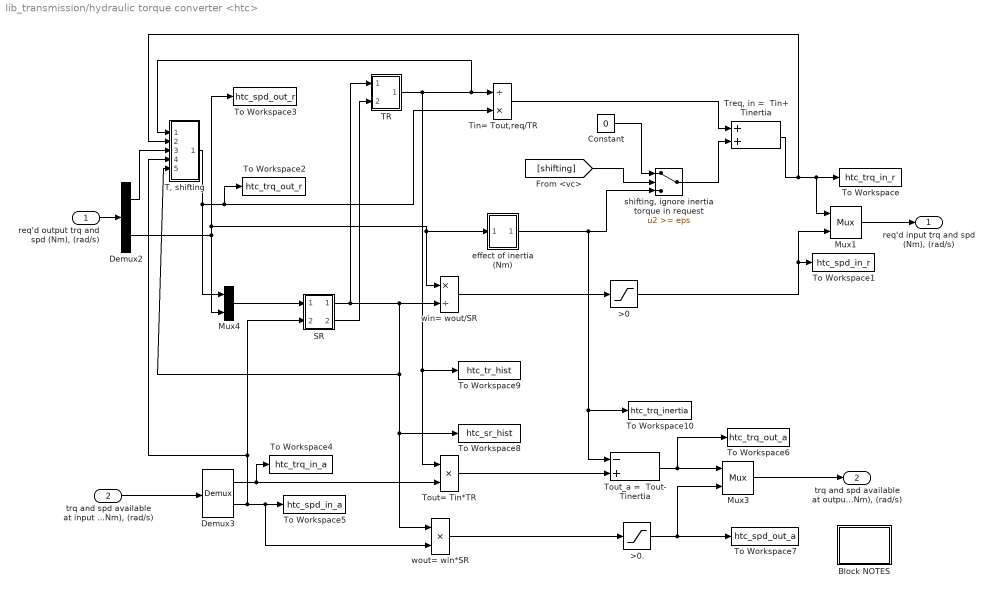
== system lib_transmission/hydraulic torque converter <htc> ==
  "req'd output trq and spd (Nm), (rad/s)" : Inport  Port=1  LatchInput=off
  "trq and spd available at input (Nm), (rad/s)" : Inport  Port=2  LatchInput=off
  ">0 " : Saturate  UpperLimit=inf  LowerLimit=0  LinearizeAsGain=on
  >0. : Saturate  UpperLimit=inf  LowerLimit=0  LinearizeAsGain=on
  Block NOTES : Subsystem
      settings: RTWFcnNameOpts=Auto  RTWFileNameOpts=Auto
      mask Display: disp('Block\nNOTES')
  Constant : Constant  Value=0
  Demux2 : Demux  Outputs=2  BusSelectionMode=off
  Demux3 : Demux  Outputs=2  BusSelectionMode=off
  Mux1 : Mux  Inputs=2
      settings: DisplayOption=none
  Mux3 : Mux  Inputs=2
      settings: DisplayOption=none
  Mux4 : Mux  Inputs=2
      settings: DisplayOption=none
  SR : Subsystem
      settings: RTWFcnNameOpts=Auto  RTWFileNameOpts=Auto
  "T, shifting" : Subsystem
      settings: RTWFcnNameOpts=Auto  RTWFileNameOpts=Auto
  TR : Subsystem
      settings: RTWFcnNameOpts=Auto  RTWFileNameOpts=Auto
  Tin= Tout,req/TR : Product  Inputs=/*  Multiplication=Element-wise(.*)  SaturateOnIntegerOverflow=on
  To Workspace : ToWorkspace  VariableName=htc_trq_in_r  SampleTime=-1  SaveFormat=Array
  To Workspace1 : ToWorkspace  VariableName=htc_spd_in_r  SampleTime=-1  SaveFormat=Array
  To Workspace10 : ToWorkspace  VariableName=htc_trq_inertia  SampleTime=-1  SaveFormat=Array
  To Workspace2 : ToWorkspace  VariableName=htc_trq_out_r  SampleTime=-1  SaveFormat=Array
  To Workspace3 : ToWorkspace  VariableName=htc_spd_out_r  SampleTime=-1  SaveFormat=Array
  To Workspace4 : ToWorkspace  VariableName=htc_trq_in_a  SampleTime=-1  SaveFormat=Array
  To Workspace5 : ToWorkspace  VariableName=htc_spd_in_a  SampleTime=-1  SaveFormat=Array
  To Workspace6 : ToWorkspace  VariableName=htc_trq_out_a  SampleTime=-1  SaveFormat=Array
  To Workspace7 : ToWorkspace  VariableName=htc_spd_out_a  SampleTime=-1  SaveFormat=Array
  To Workspace8 : ToWorkspace  VariableName=htc_sr_hist  SampleTime=-1  SaveFormat=Array
  To Workspace9 : ToWorkspace  VariableName=htc_tr_hist  SampleTime=-1  SaveFormat=Array
  Tout= Tin*TR : Product  Inputs=**  Multiplication=Element-wise(.*)  SaturateOnIntegerOverflow=on
  Tout_a =  Tout- Tinertia : Sum  Inputs=-+  SaturateOnIntegerOverflow=on
  "Treq, in =  Tin+ Tinertia" : Sum  Inputs=++  SaturateOnIntegerOverflow=on
  effect of inertia (Nm) : Subsystem
      settings: RTWFcnNameOpts=Auto  RTWFileNameOpts=Auto
  "shifting, ignore inertia torque in request" : Switch  Threshold=eps
  win= wout/SR : Product  Inputs=*/  Multiplication=Element-wise(.*)  SaturateOnIntegerOverflow=on
  wout= win*SR : Product  Inputs=**  Multiplication=Element-wise(.*)  SaturateOnIntegerOverflow=on
  "req'd input trq and spd (Nm), (rad/s)" : Outport  Port=1  InitialOutput=0
  "trq and spd available at output (Nm), (rad/s)" : Outport  Port=2  InitialOutput=0
  wires:
  >0./1 -> Mux3/2, To Workspace7/1
  wout= win*SR/1 -> >0./1
  Demux3/1 -> To Workspace4/1, Tout= Tin*TR/2
  "trq and spd available at input (Nm), (rad/s)"/1 -> Demux3/1
  Tout= Tin*TR/1 -> Tout_a =  Tout- Tinertia/2
  Mux3/1 -> "trq and spd available at output (Nm), (rad/s)"/1
  win= wout/SR/1 -> ">0 "/1
  "T, shifting"/1(T req) -> Mux4/1, Tin= Tout,req/TR/2, To Workspace2/1
  Demux2/1 -> "T, shifting"/3(Req'd output trq)
  Demux3/2 -> To Workspace5/1, wout= win*SR/2, SR/2(w in), "T, shifting"/4(htc_spd_in_a)
  Mux4/1 -> SR/1(T,w req out)
  SR/1(SR) -> win= wout/SR/2, wout= win*SR/1, To Workspace8/1, "T, shifting"/5(SR), TR/1(SR)
  Tout_a =  Tout- Tinertia/1 -> Mux3/1, To Workspace6/1
  Demux2/2 -> Mux4/2, win= wout/SR/1, effect of inertia (Nm)/1(turbine/output speed (rad/s)), To Workspace3/1
  ">0 "/1 -> To Workspace1/1, Mux1/2
  Constant/1 -> "shifting, ignore inertia torque in request"/1
  effect of inertia (Nm)/1(inertia torque (Nm)) -> Tout_a =  Tout- Tinertia/1, To Workspace10/1, "shifting, ignore inertia torque in request"/3
  TR/1(TR) -> Tout= Tin*TR/1, To Workspace9/1, Tin= Tout,req/TR/1, "T, shifting"/1(TR)
  SR/2(coasting) -> TR/2(coasting)
  Mux1/1 -> "req'd input trq and spd (Nm), (rad/s)"/1
  "Treq, in =  Tin+ Tinertia"/1 -> Mux1/1, To Workspace/1, "T, shifting"/2(Req'd  input trq)
  "shifting, ignore inertia torque in request"/1 -> "Treq, in =  Tin+ Tinertia"/2
  Tin= Tout,req/TR/1 -> "Treq, in =  Tin+ Tinertia"/1
  "req'd output trq and spd (Nm), (rad/s)"/1 -> Demux2/1
  [shifting] -> "shifting, ignore inertia torque in request"/2

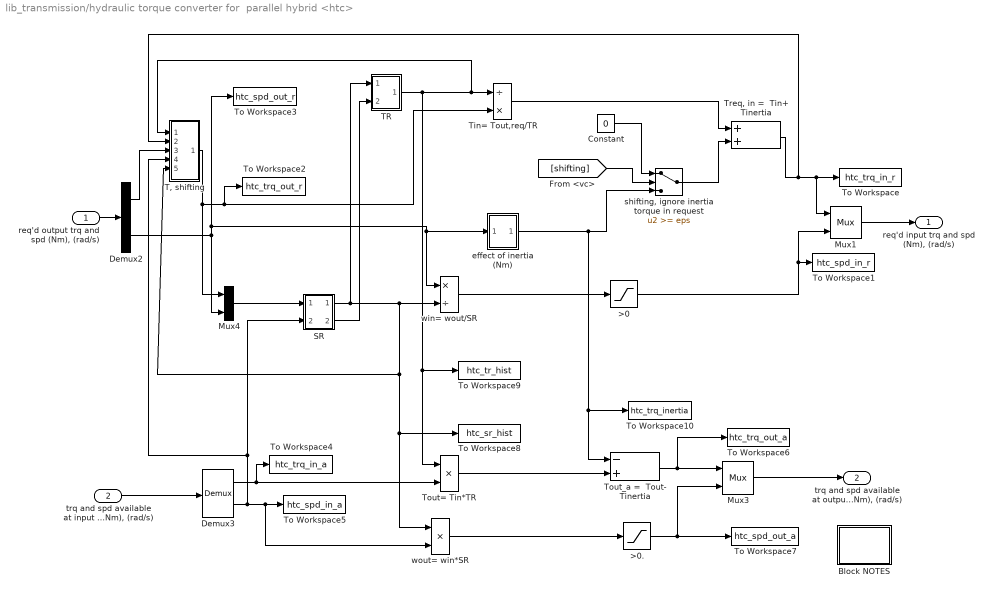
== system lib_transmission/hydraulic torque converter for  parallel hybrid <htc> ==
  "req'd output trq and spd (Nm), (rad/s)" : Inport  Port=1  LatchInput=off
  "trq and spd available at input (Nm), (rad/s)" : Inport  Port=2  LatchInput=off
  ">0 " : Saturate  UpperLimit=inf  LowerLimit=0  LinearizeAsGain=on
  >0. : Saturate  UpperLimit=inf  LowerLimit=0  LinearizeAsGain=on
  Block NOTES : Subsystem
      settings: RTWFcnNameOpts=Auto  RTWFileNameOpts=Auto
      mask Display: disp('Block\nNOTES')
  Constant : Constant  Value=0
  Demux2 : Demux  Outputs=2  BusSelectionMode=off
  Demux3 : Demux  Outputs=2  BusSelectionMode=off
  Mux1 : Mux  Inputs=2
      settings: DisplayOption=none
  Mux3 : Mux  Inputs=2
      settings: DisplayOption=none
  Mux4 : Mux  Inputs=2
      settings: DisplayOption=none
  SR : Subsystem
      settings: RTWFcnNameOpts=Auto  RTWFileNameOpts=Auto
  "T, shifting" : Subsystem
      settings: RTWFcnNameOpts=Auto  RTWFileNameOpts=Auto
  TR : Subsystem
      settings: RTWFcnNameOpts=Auto  RTWFileNameOpts=Auto
  Tin= Tout,req/TR : Product  Inputs=/*  Multiplication=Element-wise(.*)  SaturateOnIntegerOverflow=on
  To Workspace : ToWorkspace  VariableName=htc_trq_in_r  SampleTime=-1  SaveFormat=Array
  To Workspace1 : ToWorkspace  VariableName=htc_spd_in_r  SampleTime=-1  SaveFormat=Array
  To Workspace10 : ToWorkspace  VariableName=htc_trq_inertia  SampleTime=-1  SaveFormat=Array
  To Workspace2 : ToWorkspace  VariableName=htc_trq_out_r  SampleTime=-1  SaveFormat=Array
  To Workspace3 : ToWorkspace  VariableName=htc_spd_out_r  SampleTime=-1  SaveFormat=Array
  To Workspace4 : ToWorkspace  VariableName=htc_trq_in_a  SampleTime=-1  SaveFormat=Array
  To Workspace5 : ToWorkspace  VariableName=htc_spd_in_a  SampleTime=-1  SaveFormat=Array
  To Workspace6 : ToWorkspace  VariableName=htc_trq_out_a  SampleTime=-1  SaveFormat=Array
  To Workspace7 : ToWorkspace  VariableName=htc_spd_out_a  SampleTime=-1  SaveFormat=Array
  To Workspace8 : ToWorkspace  VariableName=htc_sr_hist  SampleTime=-1  SaveFormat=Array
  To Workspace9 : ToWorkspace  VariableName=htc_tr_hist  SampleTime=-1  SaveFormat=Array
  Tout= Tin*TR : Product  Inputs=**  Multiplication=Element-wise(.*)  SaturateOnIntegerOverflow=on
  Tout_a =  Tout- Tinertia : Sum  Inputs=-+  SaturateOnIntegerOverflow=on
  "Treq, in =  Tin+ Tinertia" : Sum  Inputs=++  SaturateOnIntegerOverflow=on
  effect of inertia (Nm) : Subsystem
      settings: RTWFcnNameOpts=Auto  RTWFileNameOpts=Auto
  "shifting, ignore inertia torque in request" : Switch  Threshold=eps
  win= wout/SR : Product  Inputs=*/  Multiplication=Element-wise(.*)  SaturateOnIntegerOverflow=on
  wout= win*SR : Product  Inputs=**  Multiplication=Element-wise(.*)  SaturateOnIntegerOverflow=on
  "req'd input trq and spd (Nm), (rad/s)" : Outport  Port=1  InitialOutput=0
  "trq and spd available at output (Nm), (rad/s)" : Outport  Port=2  InitialOutput=0
  wires:
  "req'd output trq and spd (Nm), (rad/s)"/1 -> Demux2/1
  Tin= Tout,req/TR/1 -> "Treq, in =  Tin+ Tinertia"/1
  "shifting, ignore inertia torque in request"/1 -> "Treq, in =  Tin+ Tinertia"/2
  "Treq, in =  Tin+ Tinertia"/1 -> "T, shifting"/2(Req'd  input trq), To Workspace/1, Mux1/1
  Mux1/1 -> "req'd input trq and spd (Nm), (rad/s)"/1
  SR/2(coasting) -> TR/2(coasting)
  TR/1(TR) -> "T, shifting"/1(TR), Tin= Tout,req/TR/1, To Workspace9/1, Tout= Tin*TR/1
  effect of inertia (Nm)/1(inertia torque (Nm)) -> "shifting, ignore inertia torque in request"/3, To Workspace10/1, Tout_a =  Tout- Tinertia/1
  Constant/1 -> "shifting, ignore inertia torque in request"/1
  ">0 "/1 -> Mux1/2, To Workspace1/1
  Demux2/2 -> To Workspace3/1, effect of inertia (Nm)/1(turbine/output speed (rad/s)), win= wout/SR/1, Mux4/2
  Tout_a =  Tout- Tinertia/1 -> To Workspace6/1, Mux3/1
  SR/1(SR) -> TR/1(SR), "T, shifting"/5(SR), To Workspace8/1, wout= win*SR/1, win= wout/SR/2
  Mux4/1 -> SR/1(T,w req out)
  Demux3/2 -> "T, shifting"/4(htc_spd_in_a), SR/2(w in), wout= win*SR/2, To Workspace5/1
  Demux2/1 -> "T, shifting"/3(Req'd output trq)
  "T, shifting"/1(T req) -> To Workspace2/1, Tin= Tout,req/TR/2, Mux4/1
  win= wout/SR/1 -> ">0 "/1
  Mux3/1 -> "trq and spd available at output (Nm), (rad/s)"/1
  Tout= Tin*TR/1 -> Tout_a =  Tout- Tinertia/2
  "trq and spd available at input (Nm), (rad/s)"/1 -> Demux3/1
  Demux3/1 -> Tout= Tin*TR/2, To Workspace4/1
  wout= win*SR/1 -> >0./1
  >0./1 -> To Workspace7/1, Mux3/2
  [shifting] -> "shifting, ignore inertia torque in request"/2

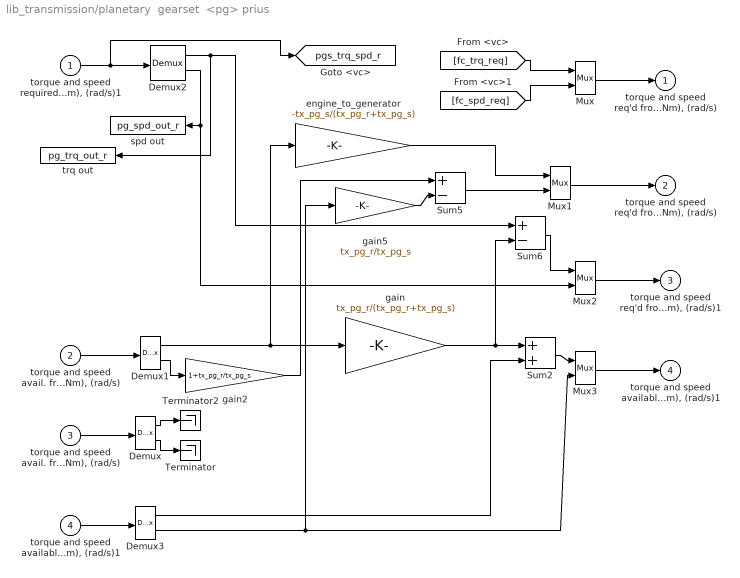
== system lib_transmission/planetary  gearset  <pg> prius ==
  "torque and speed required from ring gear (Nm), (rad/s)1" : Inport  Port=1  LatchInput=off
  "torque and speed avail. from fuel converter (Nm), (rad/s)" : Inport  Port=2  LatchInput=off
  "torque and speed avail. from generator (Nm), (rad/s)" : Inport  Port=3  LatchInput=off
  "torque and speed available from motor (Nm), (rad/s)1" : Inport  Port=4  LatchInput=off
  Demux{,1..3} (4 alike) : Demux  Outputs=2  BusSelectionMode=off
  Mux{,1..3} (4 alike) : Mux  Inputs=2
      settings: DisplayOption=none
  Sum2 : Sum  Inputs=++  SaturateOnIntegerOverflow=on
  Sum5 : Sum  Inputs=+-  SaturateOnIntegerOverflow=on
  Sum6 : Sum  Inputs=+-  SaturateOnIntegerOverflow=on
  Terminator : Terminator
  Terminator2 : Terminator
  engine_to_generator : Gain  Gain=-tx_pg_s/(tx_pg_r+tx_pg_s)  Multiplication=Element-wise(K.*u)  SaturateOnIntegerOverflow=on
  gain : Gain  Gain=tx_pg_r/(tx_pg_r+tx_pg_s)  Multiplication=Element-wise(K.*u)  SaturateOnIntegerOverflow=on
  gain2 : Gain  Gain=1+tx_pg_r/tx_pg_s  Multiplication=Element-wise(K.*u)  SaturateOnIntegerOverflow=on
  gain5 : Gain  Gain=tx_pg_r/tx_pg_s  Multiplication=Element-wise(K.*u)  SaturateOnIntegerOverflow=on
  spd out : ToWorkspace  VariableName=pg_spd_out_r  SampleTime=0  SaveFormat=Array
      settings: MaxDataPoints=100000
  trq out : ToWorkspace  VariableName=pg_trq_out_r  SampleTime=0  SaveFormat=Array
      settings: MaxDataPoints=100000
  "torque and speed req'd from fuel converter (Nm), (rad/s)" : Outport  Port=1  InitialOutput=0
  "torque and speed req'd from generator (Nm), (rad/s)" : Outport  Port=2  InitialOutput=0
  "torque and speed req'd from motor (Nm), (rad/s)1" : Outport  Port=3  InitialOutput=0
  "torque and speed available to final drive (Nm), (rad/s)1" : Outport  Port=4  InitialOutput=0
  tag scope: pgs_trq_spd_r=global
  wires:
  "torque and speed available from motor (Nm), (rad/s)1"/1 -> Demux3/1
  Demux3/2 -> gain5/1, Mux3/2
  Demux3/1 -> Sum2/2
  Mux3/1 -> "torque and speed available to final drive (Nm), (rad/s)1"/1
  Sum2/1 -> Mux3/1
  Sum5/1 -> Mux1/2
  engine_to_generator/1 -> Mux1/1
  Mux1/1 -> "torque and speed req'd from generator (Nm), (rad/s)"/1
  Sum6/1 -> Mux2/1
  Mux2/1 -> "torque and speed req'd from motor (Nm), (rad/s)1"/1
  gain2/1 -> Sum5/1
  Demux/2 -> Terminator/1
  Demux/1 -> Terminator2/1
  "torque and speed avail. from generator (Nm), (rad/s)"/1 -> Demux/1
  Demux1/1 -> engine_to_generator/1, gain/1
  Demux1/2 -> gain2/1
  "torque and speed avail. from fuel converter (Nm), (rad/s)"/1 -> Demux1/1
  gain5/1 -> Sum5/2
  [fc_trq_req] -> Mux/1
  [fc_spd_req] -> Mux/2
  Mux/1 -> "torque and speed req'd from fuel converter (Nm), (rad/s)"/1
  Demux2/1 -> Sum6/1, trq out/1
  Demux2/2 -> Mux2/2, spd out/1
  gain/1 -> Sum2/1, Sum6/2
  "torque and speed required from ring gear (Nm), (rad/s)1"/1 -> [pgs_trq_spd_r], Demux2/1

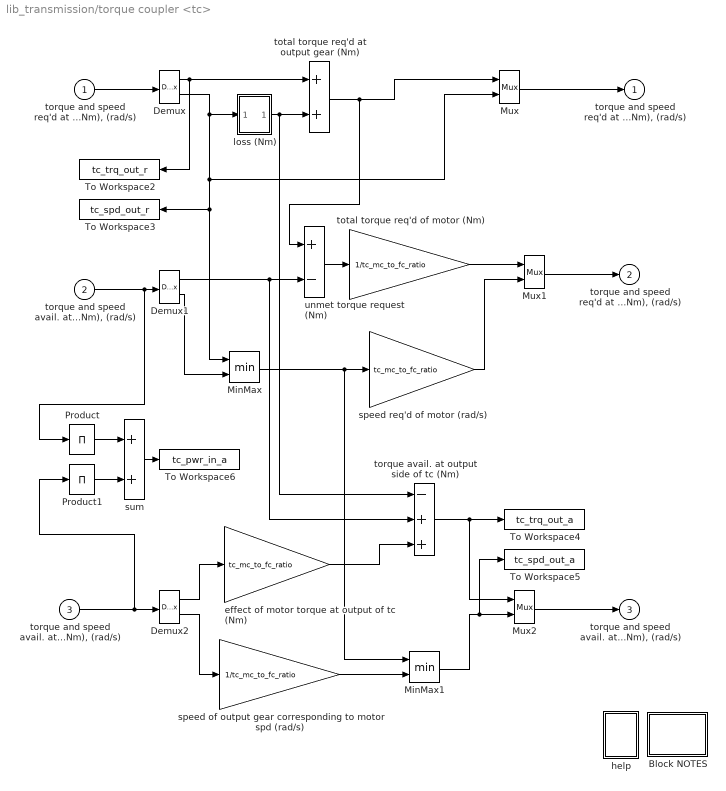
== system lib_transmission/torque coupler <tc> ==
  "torque and speed req'd at output side of torque coupler (Nm), (rad/s)" : Inport  Port=1  LatchInput=off
  "torque and speed avail. at main input (Nm), (rad/s)" : Inport  Port=2  LatchInput=off
  "torque and speed avail. at motor input to tc (Nm), (rad/s)" : Inport  Port=3  LatchInput=off
  Block NOTES : Subsystem
      settings: RTWFcnNameOpts=Auto  RTWFileNameOpts=Auto
      mask Display: disp('Block\nNOTES')
  Demux : Demux  Outputs=2  BusSelectionMode=off
  Demux1 : Demux  Outputs=2  BusSelectionMode=off
  Demux2 : Demux  Outputs=2  BusSelectionMode=off
  MinMax : MinMax  Function=min  Inputs=2
  MinMax1 : MinMax  Function=min  Inputs=2
  Mux : Mux  Inputs=2
      settings: DisplayOption=none
  Mux1 : Mux  Inputs=2
      settings: DisplayOption=none
  Mux2 : Mux  Inputs=2
      settings: DisplayOption=none
  Product : Product  Inputs=1  Multiplication=Element-wise(.*)  SaturateOnIntegerOverflow=on
  Product1 : Product  Inputs=1  Multiplication=Element-wise(.*)  SaturateOnIntegerOverflow=on
  To Workspace2 : ToWorkspace  VariableName=tc_trq_out_r  SampleTime=-1  SaveFormat=Array
  To Workspace3 : ToWorkspace  VariableName=tc_spd_out_r  SampleTime=-1  SaveFormat=Array
  To Workspace4 : ToWorkspace  VariableName=tc_trq_out_a  SampleTime=-1  SaveFormat=Array
  To Workspace5 : ToWorkspace  VariableName=tc_spd_out_a  SampleTime=-1  SaveFormat=Array
  To Workspace6 : ToWorkspace  VariableName=tc_pwr_in_a  SampleTime=-1  SaveFormat=Array
  effect of motor torque at output of tc (Nm) : Gain  Gain=tc_mc_to_fc_ratio  Multiplication=Element-wise(K.*u)  SaturateOnIntegerOverflow=on
  help : Subsystem
      settings: OpenFcn=web(['file:\\\' which('torque_coupler.htm')]);  RTWFcnNameOpts=Auto  RTWFileNameOpts=Auto
      mask Display: image(imread('doc_man.jpg'))
  loss (Nm) : Subsystem
      settings: RTWFcnNameOpts=Auto  RTWFileNameOpts=Auto
  speed of output gear corresponding to motor spd (rad/s) : Gain  Gain=1/tc_mc_to_fc_ratio  Multiplication=Element-wise(K.*u)  SaturateOnIntegerOverflow=on
  speed req'd of motor (rad/s) : Gain  Gain=tc_mc_to_fc_ratio  Multiplication=Element-wise(K.*u)  SaturateOnIntegerOverflow=on
  "sum " : Sum  Inputs=++  SaturateOnIntegerOverflow=on
  torque avail. at output side of tc (Nm) : Sum  Inputs=-++  SaturateOnIntegerOverflow=on
  total torque req'd at output gear (Nm) : Sum  Inputs=++  SaturateOnIntegerOverflow=on
  total torque req'd of motor (Nm) : Gain  Gain=1/tc_mc_to_fc_ratio  Multiplication=Element-wise(K.*u)  SaturateOnIntegerOverflow=on
  unmet torque request (Nm) : Sum  Inputs=+-  SaturateOnIntegerOverflow=on
  "torque and speed req'd at main input to torque coupler (Nm), (rad/s)" : Outport  Port=1  InitialOutput=0
  "torque and speed req'd at motor input to torque coupler (Nm), (rad/s)" : Outport  Port=2  InitialOutput=0
  "torque and speed avail. at output side of torque coupler (Nm), (rad/s)" : Outport  Port=3  InitialOutput=0
  wires:
  MinMax1/1 -> To Workspace5/1, Mux2/2
  torque avail. at output side of tc (Nm)/1 -> To Workspace4/1, Mux2/1
  Demux/1 -> To Workspace2/1, total torque req'd at output gear (Nm)/1
  MinMax/1 -> MinMax1/1, speed req'd of motor (rad/s)/1
  speed of output gear corresponding to motor spd (rad/s)/1 -> MinMax1/2
  Demux2/2 -> speed of output gear corresponding to motor spd (rad/s)/1
  Mux2/1 -> "torque and speed avail. at output side of torque coupler (Nm), (rad/s)"/1
  effect of motor torque at output of tc (Nm)/1 -> torque avail. at output side of tc (Nm)/3
  Demux2/1 -> effect of motor torque at output of tc (Nm)/1
  Demux1/1 -> torque avail. at output side of tc (Nm)/2, unmet torque request (Nm)/2
  loss (Nm)/1(drag torque (Nm)) -> torque avail. at output side of tc (Nm)/1, total torque req'd at output gear (Nm)/2
  speed req'd of motor (rad/s)/1 -> Mux1/2
  total torque req'd of motor (Nm)/1 -> Mux1/1
  Mux1/1 -> "torque and speed req'd at motor input to torque coupler (Nm), (rad/s)"/1
  Demux1/2 -> MinMax/2
  unmet torque request (Nm)/1 -> total torque req'd of motor (Nm)/1
  total torque req'd at output gear (Nm)/1 -> unmet torque request (Nm)/1, Mux/1
  Demux/2 -> To Workspace3/1, MinMax/1, Mux/2, loss (Nm)/1(tc output speed (rad/s))
  "torque and speed req'd at output side of torque coupler (Nm), (rad/s)"/1 -> Demux/1
  Mux/1 -> "torque and speed req'd at main input to torque coupler (Nm), (rad/s)"/1
  "sum "/1 -> To Workspace6/1
  Product/1 -> "sum "/1
  "torque and speed avail. at main input (Nm), (rad/s)"/1 -> Demux1/1, Product/1
  "torque and speed avail. at motor input to tc (Nm), (rad/s)"/1 -> Demux2/1, Product1/1
  Product1/1 -> "sum "/2
